simulink model "s_aero_2dof_lqr_control"  (R2016a)
settings: Solver=ode1  StartTime=0.0  StopTime=30  FixedStep=0.002  RelTol=1e-3
values from neighbouring files (symbols this model uses):
  A = [0 0 1 0 ... (first row only)    [ONline.m]
  B = [0 0 ... (first row only)    [ONline.m]
undefined symbols (not defined in the file or in its folder): C, D
libraries: simulink_extras x4, quarc_library x3
settings Model: ExtModeTrigDuration=5000  Creator=MLevis  LastModifiedBy=anc
settings SolverCC: PositivePriorityOrder=on
settings DataIOCC: LimitDataPoints=on  SaveFormat=Array
settings DebuggingCC: SolverPrmCheckMsg=warning
settings HardwareCC: ProdBitPerPointer=32  ProdLargestAtomicFloat=None  ProdIntDivRoundTo=Undefined  ProdEndianess=Unspecified  ProdWordSize=32  ProdHWDeviceType=32-bit Generic
settings ModelReferenceCC: PropagateSignalLabelsOutOfModel=off
settings RTWCC: SystemTargetFile=quarc_win64.tlc  TemplateMakefile=quarc_default_tmf  Description=QUARC Win64 Target
settings STFCustomTargetCC: TargetPreCompLibLocation=C:\PROGRA~3\QUARC\lib\2016a\win64\release  ConcurrentExecutionCompliant=on  GeneratePreprocessorConditionals=Disable all  SystemTargetFile=quarc_win64.tlc
settings GRTTargetCC: TargetPreCompLibLocation=C:\PROGRA~3\QUARC\lib\2016a\win64\release  ParMdlRefBuildCompliant=off  CompOptLevelCompliant=off  CombineOutputUpdateFcns=off  MatFileLogging=off  CPPClassGenCompliant=off  GRTInterface=on  UseToolchainInfoCompliant=off  ExtMode=on  ExtModeMexFile=quarc_comm
settings ConfigComp: CovModelRefEnable=Off  CovSFcnEnable=off

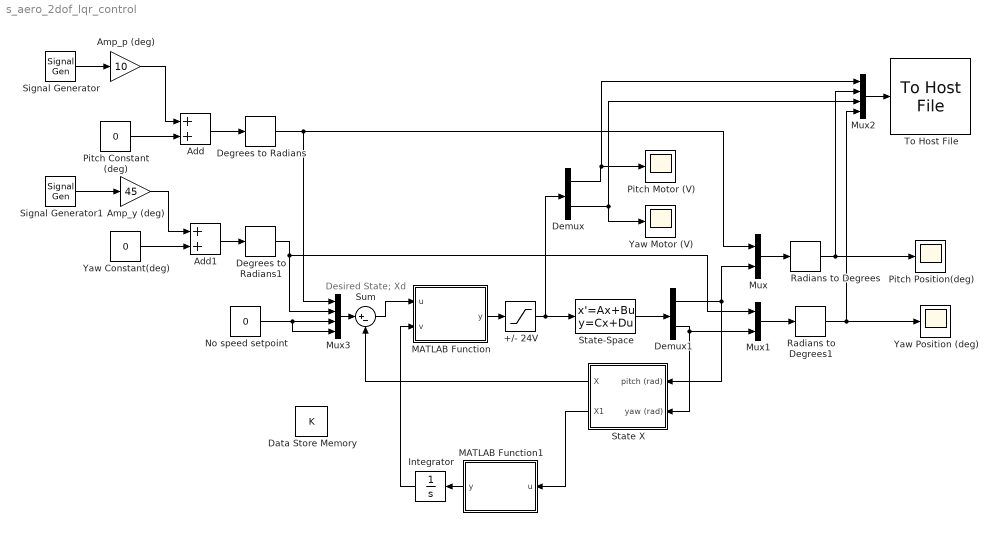
== system s_aero_2dof_lqr_control ==
  note: Desired State; Xd
  +/- 24V : Saturate  UpperLimit=24  LowerLimit=-24
  Add : Sum
  Add1 : Sum
  Amp_p (deg) : Gain  Gain=10
  Amp_y (deg) : Gain  Gain=45
  Data Store Memory : DataStoreMemory  DataStoreName=K  ReadBeforeWriteMsg=warning  WriteAfterWriteMsg=warning  WriteAfterReadMsg=warning  InitialValue=[90 -100 30 -30;150 50 40 15]  ShowAdditionalParam=off  OutDataTypeStr=double
  Degrees to Radians : simulink_extras/Transformations/Degrees to Radians
  Degrees to Radians1 : simulink_extras/Transformations/Degrees to Radians
  Demux : Demux  Outputs=2
  Demux1 : Demux  Outputs=2
  Integrator : Integrator
  MATLAB Function : MATLAB Function  TreatAsAtomicUnit=on
  MATLAB Function1 : MATLAB Function  TreatAsAtomicUnit=on
  Mux : Mux  Inputs=2
  Mux1 : Mux  Inputs=2
  Mux2 : Mux
  Mux3 : Mux
  No speed setpoint : Constant  Value=0
  Pitch Constant (deg) : Constant  Value=0
  Pitch Motor (V) : Scope
  Pitch Position(deg) : Scope
  Radians to Degrees : simulink_extras/Transformations/Radians to Degrees
  Radians to Degrees1 : simulink_extras/Transformations/Radians to Degrees
  Signal Generator : SignalGenerator  WaveForm=square  Frequency=0.2
  Signal Generator1 : SignalGenerator  WaveForm=square  Frequency=0.2
  State X : Subsystem
  State-Space : StateSpace  A=A  B=B  C=C  D=D  X0=0
  Sum : Sum  Inputs=|+-
  To Host File : quarc_library/Sinks/To Host/To Host File  file_name=aero_lqr_rsp_sim.mat  variable_name=lqr_rsp_sim  decimation=1  sample_time=-1  file_format=MAT-file v.4  options=No header or footer  append=off  final_file_name=aero_lqr_rsp_sim.mat  bitrate=2000000
  Yaw Constant(deg) : Constant  Value=0
  Yaw Motor (V) : Scope
  Yaw Position (deg) : Scope
  wires:
  Degrees to Radians/1 -> Mux3/1, Mux/1
  Degrees to Radians1/1 -> Mux3/2, Mux1/1
  Signal Generator/1 -> Amp_p (deg)/1
  Pitch Constant (deg)/1 -> Add/2
  Add/1 -> Degrees to Radians/1
  Yaw Constant(deg)/1 -> Add1/2
  Signal Generator1/1 -> Amp_y (deg)/1
  Add1/1 -> Degrees to Radians1/1
  Mux/1 -> Radians to Degrees/1
  Radians to Degrees/1 -> Mux2/2, Pitch Position(deg)/1
  Radians to Degrees1/1 -> Mux2/4, Yaw Position (deg)/1
  Demux/1 -> Mux2/1, Pitch Motor (V)/1
  Demux/2 -> Yaw Motor (V)/1, Mux2/3
  Mux1/1 -> Radians to Degrees1/1
  Mux3/1 -> Sum/1
  No speed setpoint/1 -> Mux3/4, Mux3/3
  +/- 24V/1 -> State-Space/1, Demux/1
  State X/1(X) -> Sum/2
  Demux1/1 -> Mux/2, State X/1(pitch (rad))
  State-Space/1 -> Demux1/1
  Demux1/2 -> Mux1/2, State X/2(yaw (rad))
  Mux2/1 -> To Host File/1
  MATLAB Function/1(y) -> +/- 24V/1
  Amp_p (deg)/1 -> Add/1
  Amp_y (deg)/1 -> Add1/1
  Sum/1 -> MATLAB Function/1(u)
  MATLAB Function1/1(y) -> Integrator/1
  Integrator/1 -> MATLAB Function/2(v)
  State X/2(X1) -> MATLAB Function1/1(u)

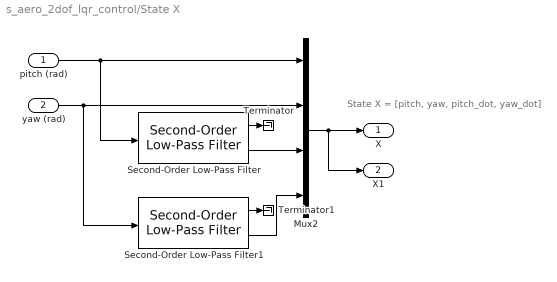
== system s_aero_2dof_lqr_control/State X ==
  note: State X = [pitch, yaw, pitch_dot, yaw_dot]
  pitch (rad) : Inport
  yaw (rad) : Inport  Port=2
  Mux2 : Mux
  Second-Order Low-Pass Filter : quarc_library/Continuous/Second-Order Low-Pass Filter  params_source=Internal (dialog parameters)  input_width=50  input_zeta=0.8  input_init=0
  Second-Order Low-Pass Filter1 : quarc_library/Continuous/Second-Order Low-Pass Filter  params_source=Internal (dialog parameters)  input_width=50  input_zeta=0.8  input_init=0
  Terminator : Terminator
  Terminator1 : Terminator
  X : Outport
  X1 : Outport  Port=2
  wires:
  yaw (rad)/1 -> Second-Order Low-Pass Filter1/1, Mux2/2
  pitch (rad)/1 -> Second-Order Low-Pass Filter/1, Mux2/1
  Second-Order Low-Pass Filter/2 -> Mux2/3
  Second-Order Low-Pass Filter1/2 -> Mux2/4
  Second-Order Low-Pass Filter/1 -> Terminator/1
  Second-Order Low-Pass Filter1/1 -> Terminator1/1
  Mux2/1 -> X1/1, X/1

== matlab function s_aero_2dof_lqr_control/MATLAB Function1 ==
  data: u input; y output; K data_store_memory
function y = fcn(u)
%#codegen
global K ;

Q = diag([200 75 0 0]) ;
R = 0.005 * eye(2,2) ;

%x_1 = [u(1) u(2) u(3) u(4)]' ;

out = u' * (Q + K'*R*K) * u ;
y=zeros(1,1) ;

y = out ;

== matlab function s_aero_2dof_lqr_control/MATLAB Function ==
  data: u input; v input; y output; K data_store_memory
function y = fcn(u, v)

global K ;

%to find the optimal feedback control law k.
%K = zeros(2, 4) ;

% this is similar to the optimal control gain
%    98.2088 -103.0645   32.2643  -29.0750
%   156.3469   66.1643   45.5122   17.1068
% K = [90 -100   30  -30;
%       150   50   40   15] ;
  
B = [0 0;                 
    0 0;
    0.0503 0.0959;
    -0.1228 0.1] ;

% Q = diag([200 75 0 0]) ;
R = 0.005 * eye(2,2) ;

dT = 0.05 ;     % sampe interval
T = 20 ;        % samp nums
X = zeros(10, T) ;
Y = zeros(T, 1) ;

for i = 1 : T
    x_t = [u(1) u(2) u(3) u(4)] ; 
    v_t = v ;
    %delay(dT) ;     % how to delay 0.05s?
    for m=1:1:25
        
    end
    x_T = [u(1) u(2) u(3) u(4)] ;
    
    %v = dT * ((x_t+x_T)/2) * (Q+K'*R*K) * ((x_t+x_T)/2)' ;
    v_T = v ;
    
    % cal the Kronecker product of x
    nums = 1 ;
    bar_x_t = zeros(10, 1) ;
    bar_x_T = zeros(10, 1) ;
    for temp1 = 1 : 4
        for temp2 = temp1 : 4
            bar_x_t(nums) = x_t(temp1) * x_t(temp2) ;
            bar_x_T(nums) = x_T(temp1) * x_T(temp2) ;
            nums = nums + 1 ;
        end
    end

    delta_x = bar_x_t - bar_x_T ;
    X(1:10, i) = delta_x ;      
    Y(i, 1) = v_T - v_t ;
end

%bar_p = inv(X*X')*X*Y ;
bar_p = X'\Y ;

P = [bar_p(1) bar_p(2)/2 bar_p(3)/2 bar_p(4)/2;
     bar_p(2)/2 bar_p(5) bar_p(6)/2 bar_p(7)/2;
     bar_p(3)/2 bar_p(6)/2 bar_p(8) bar_p(9)/2;
     bar_p(4)/2 bar_p(7)/2 bar_p(9)/2 bar_p(10)] ;

K = R\B' * P ;

y = -K *  x_T' ;
